simulink model "CanSat"  (Simulink 7.3)
settings: Solver=ode45  StartTime=0.0  StopTime=2  RelTol=1e-3
undefined symbols (not defined in the file or in its folder): DiscIntNeverNeededParam
settings Model: Creator=Sainquake Notebook  LastModifiedBy=Sainquake

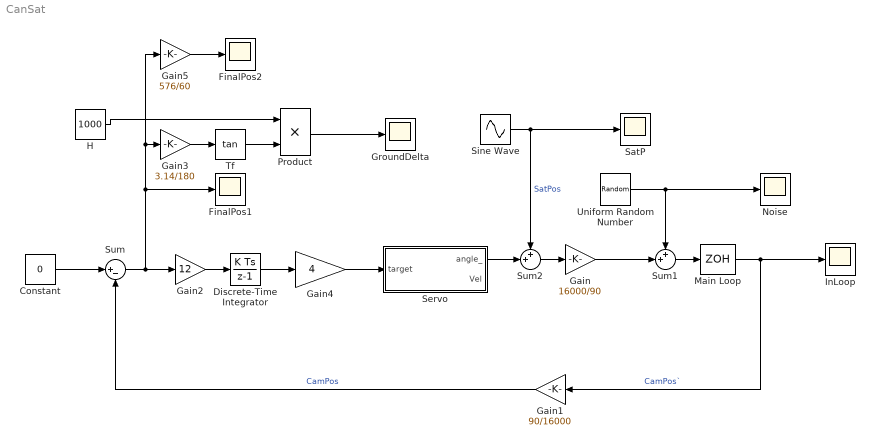
== system CanSat ==
  Constant : Constant  Value=0  OutDataType=fixdt(1, 16)  OutScaling=2^0
  Discrete-Time Integrator : DiscreteIntegrator  SampleTime=0.0001  OutDataType=fixdt(1, 16)  OutScaling=2^0  ICPrevOutput=DiscIntNeverNeededParam  ICPrevScaledInput=DiscIntNeverNeededParam
  FinalPos1 : Scope
      settings: SaveName=ScopeData4  MaxDataPoints=50000
  FinalPos2 : Scope
      settings: SaveName=ScopeData8  MaxDataPoints=50000
  Gain : Gain  Gain=16000/90  ParameterDataType=fixdt(1, 16)  ParameterScaling=2^0  OutDataType=fixdt(1, 16)  OutScaling=2^0
  Gain1 : Gain  Gain=90/16000  ParameterDataType=fixdt(1, 16)  ParameterScaling=2^0  OutDataType=fixdt(1, 16)  OutScaling=2^0
  Gain2 : Gain  Gain=12  ParameterDataType=fixdt(1, 16)  ParameterScaling=2^0  OutDataType=fixdt(1, 16)  OutScaling=2^0
  Gain3 : Gain  Gain=3.14/180  ParameterDataType=fixdt(1, 16)  ParameterScaling=2^0  OutDataType=fixdt(1, 16)  OutScaling=2^0
  Gain4 : Gain  Gain=4  ParameterDataType=fixdt(1, 16)  ParameterScaling=2^0  OutDataType=fixdt(1, 16)  OutScaling=2^0
  Gain5 : Gain  Gain=576/60  ParameterDataType=fixdt(1, 16)  ParameterScaling=2^0  OutDataType=fixdt(1, 16)  OutScaling=2^0
  GroundDelta : Scope
      settings: SaveName=ScopeData6  MaxDataPoints=50000
  H : Constant  Value=1000  OutDataType=fixdt(1, 16)  OutScaling=2^0
  InLoop : Scope
      settings: SaveName=ScopeData3  MaxDataPoints=50000
  Main Loop : ZeroOrderHold  SampleTime=0.0001
  Noise : Scope
      settings: SaveName=ScopeData7  MaxDataPoints=50000
  Product : Product  OutDataType=fixdt(1, 16)  OutScaling=2^0  RndMeth=Zero
  SatP : Scope
      settings: SaveName=ScopeData5  MaxDataPoints=50000
  Servo : Subsystem
  Sine Wave : Sin  Amplitude=20  Bias=0  Frequency=sqrt(9.81/0.5)  Phase=0  Samples=10  SampleTime=0  Offset=0
  Sum : Sum  Inputs=|+-  OutDataType=fixdt(1, 16)  OutScaling=2^0
  Sum1 : Sum  Inputs=++|  OutDataType=fixdt(1, 16)  OutScaling=2^0
  Sum2 : Sum  Inputs=++|  OutDataType=fixdt(1, 16)  OutScaling=2^0
  Tf : Trigonometry  Operator=tan
  Uniform Random Number : UniformRandomNumber  Minimum=-300  Maximum=300  SampleTime=0.001
  wires:
  Sum/1 -> Gain2/1, FinalPos1/1, Gain3/1, Gain5/1
  Main Loop/1 -> InLoop/1, Gain1/1  "CamPos`"
  Gain1/1 -> Sum/2  "CamPos"
  Gain2/1 -> Discrete-Time Integrator/1
  Sum2/1 -> Gain/1
  Sine Wave/1 -> Sum2/1, SatP/1  "SatPos"
  Constant/1 -> Sum/1
  Servo/1(angle_) -> Sum2/2
  Gain/1 -> Sum1/2
  Discrete-Time Integrator/1 -> Gain4/1
  Sum1/1 -> Main Loop/1
  Uniform Random Number/1 -> Noise/1, Sum1/1
  Gain4/1 -> Servo/1(target)
  H/1 -> Product/1
  Tf/1 -> Product/2
  Product/1 -> GroundDelta/1
  Gain3/1 -> Tf/1
  Gain5/1 -> FinalPos2/1

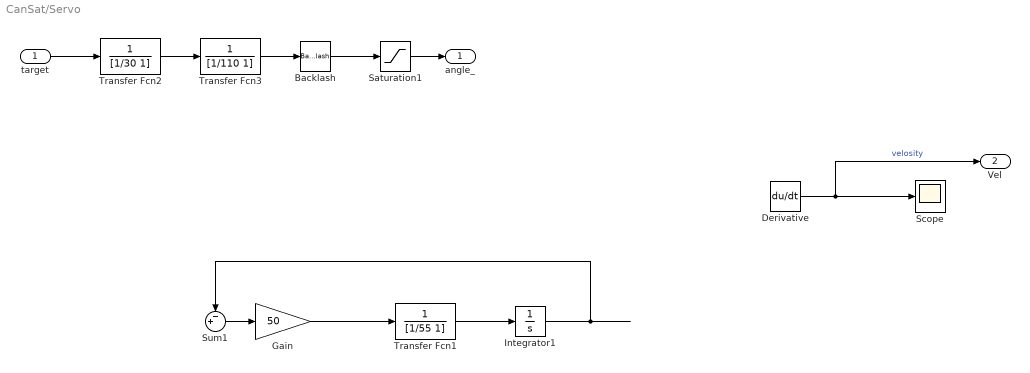
== system CanSat/Servo ==
  target : Inport  OutDataType=fixdt(1, 16)  OutScaling=2^0
  Backlash : Backlash  BacklashWidth=2
  Derivative : Derivative
  Gain : Gain  Gain=50  ParameterDataType=fixdt(1, 16)  ParameterScaling=2^0  OutDataType=fixdt(1, 16)  OutScaling=2^0
  Integrator1 : Integrator
  Saturation1 : Saturate  UpperLimit=90  LowerLimit=-90  OutDataType=fixdt(1, 16)  OutScaling=2^0
  Scope : Scope
  Sum1 : Sum  Inputs=-+|  OutDataType=fixdt(1, 16)  OutScaling=2^0
  Transfer Fcn1 : TransferFcn  Denominator=[1/55 1]
  Transfer Fcn2 : TransferFcn  Denominator=[1/30 1]
  Transfer Fcn3 : TransferFcn  Denominator=[1/110 1]
  angle_ : Outport  OutDataType=fixdt(1, 16)  OutScaling=2^0
  Vel : Outport  Port=2  OutDataType=fixdt(1, 16)  OutScaling=2^0
  wires:
  Derivative/1 -> Scope/1, Vel/1  "velosity"
  Gain/1 -> Transfer Fcn1/1
  Sum1/1 -> Gain/1
  ? -> Sum1/2
  Integrator1/1 -> Sum1/1
  Transfer Fcn1/1 -> Integrator1/1
  ? -> Derivative/1
  ? -> ?
  target/1 -> Transfer Fcn2/1
  Transfer Fcn2/1 -> Transfer Fcn3/1
  Transfer Fcn3/1 -> Backlash/1
  Backlash/1 -> Saturation1/1
  Saturation1/1 -> angle_/1
